simulink model "UAM_Flight_control"  (R2024b)
settings: Solver=FixedStepAuto  StartTime=0.0  StopTime=inf  RelTol=1e-3  EnableMultiTasking=on
undefined symbols (not defined in the file): CityMission, control, controlParams, ControlSampleTime, Cruise_a, DiscIntNeverNeededParam, Earth, FixedWingMission, flightState, FSState, FWControlParams, FWTrimSpeed, HoverMission, params, position, R_WAYPOINTTRANSITION, TransitionMission, uavParam, Vt, w_trim, WGS84, zGround
libraries: slpidlib x56, simulink x32, uavalgslib x7, robotcorelib x2, simulink_extras x2, mspfiltlib x1, aerolibtransform2 x1
(part 13 of 13)

== matlab function UAM_Flight_control/Controller/Auto1/Multicopter Controller/Attitude & Altitude controller/Altitude Control/MATLAB Function ==
  data: thrust_in input; vz input; az input; hover_est output; active input
  function hover_est = hover_thrust_lpf(thrust_in, vz, az, active)                                                  
      %#codegen                                            
      persistent hover_thrust                              
                                                           
      % Constants                                          
      HOVER_MIN = 0.2;                                     
      HOVER_MAX = 0.8;                                     
      SLEW_RATE = 0.0005;  % 200Hz 기준, 초당 0.1 변화     
      GRAVITY = 9.81;                                      
                                                           
      % Thresholds                                         
      VZ_LIM = 0.5;   % m/s                                
      AZ_LIM = 1.0;   % m/s²                               
                                                           
      if isempty(hover_thrust)                             
          hover_thrust = 0.5;                              
      end                                                  
                                                           
      hover_est = hover_thrust;                            
                                                           
      % 중력 제거                                          
      az_compensated = az + GRAVITY;                       
                                                           
      % 안정 조건 체크                                     
      is_stable = (abs(vz) < VZ_LIM) && (abs(az_compensated) < AZ_LIM);                          
                                                           
      if active && is_stable                               
          err = thrust_in - hover_thrust;                  
                                                           
          if err > SLEW_RATE                               
              hover_thrust = hover_thrust + SLEW_RATE;     
          elseif err < -SLEW_RATE                          
              hover_thrust = hover_thrust - SLEW_RATE;     
          else                                             
              hover_thrust = thrust_in;                    
          end                                              
                                                           
          hover_thrust = max(HOVER_MIN, min(HOVER_MAX, hover_thrust));                                          
      end                                                  
  end

== matlab function UAM_Flight_control/Controller/Auto1/Multicopter Controller/Attitude & Altitude controller/Derivative Gain/MATLAB Function ==
  data: x input; y output
function y = wrapToPi(x)
% x : angle error (rad)
% y : wrapped to [-pi, pi]
y = atan2(sin(x), cos(x));

== matlab function UAM_Flight_control/Controller/Auto1/Scheduler/Subsystem/Switch Case Action Subsystem/Desaturation ==
  data: m_in input; m_out output; mixMat input
function m_out = desat_px4(m_in, mixMat)
% PX4-style desaturation (MC_AIRMODE = 1, Roll/Pitch airmode)

m = m_in(:);
[N, cols] = size(mixMat);
assert(numel(m)==N && cols==4, 'mixMat must be [Nm x 4]');

act_min = zeros(N,1);
act_max = ones(N,1);
MINIMUM_YAW_MARGIN = 0.15;

thrust_z = mixMat(:,1);
roll_vec  = mixMat(:,2); %#ok<NASGU>
pitch_vec = mixMat(:,3); %#ok<NASGU>
yaw_vec   = mixMat(:,4);

% 1) thrust axis (airmode: up/down 둘 다 허용)
m = desat_axis(m, thrust_z, act_min, act_max, false);

% 2) roll/pitch는 따로 줄이지 않음 (RP airmode: 자세 우선)

% 3) yaw with margin (mixYaw()와 동일 개념)
act_max_yaw = act_max + (act_max - act_min) * MINIMUM_YAW_MARGIN;
m = desat_axis(m, yaw_vec, act_min, act_max_yaw, false);

% 4) thrust again (only down, 0~1 안으로)
m = desat_axis(m, thrust_z, act_min, act_max, true);

m_out = max(act_min, min(act_max, m));
end

function m = desat_axis(m, dir, act_min, act_max, thrust_only_down)
    k = compute_gain(dir, m, act_min, act_max);
    if ~(thrust_only_down && k > 0)
        m = m + k * dir;
    end

    k = 0.5 * compute_gain(dir, m, act_min, act_max);
    if ~(thrust_only_down && k > 0)
        m = m + k * dir;
    end
end

function k = compute_gain(dir, m, act_min, act_max)
    k_min = 0.0;
    k_max = 0.0;

    for i = 1:numel(m)
        if abs(dir(i)) < 0.2
            continue;
        end

        if m(i) < act_min(i)
            ki = (act_min(i) - m(i)) / dir(i);
            k_min = min(k_min, ki);
            k_max = max(k_max, ki);
        end

        if m(i) > act_max(i)
            ki = (act_max(i) - m(i)) / dir(i);
            k_min = min(k_min, ki);
            k_max = max(k_max, ki);
        end
    end

    k = k_min + k_max;
end

== matlab function UAM_Flight_control/Sensor/MATLAB Function6 ==
  data: YPR_raw input; YPR_corrected output; arm input
function YPR_corrected = IMU_Bias_Correction(YPR_raw, arm)
%#codegen

% Persistent variable to store bias
persistent ypr_bias;
persistent armed_prev;

if isempty(ypr_bias)
    ypr_bias = zeros(3,1);
    armed_prev = 0;
end

% Capture bias on rising edge of arm signal
if arm >= 1 && armed_prev < 1
    ypr_bias = YPR_raw;
end

armed_prev = arm;

% Apply bias correction
YPR_corrected = YPR_raw - ypr_bias;
